simulink subsystem "subsystem_feedbackLinearization"  (R2022a)
settings: Solver=VariableStepAuto  StartTime=0.0  StopTime=10.0  RelTol=1e-3
settings Model: Creator=Philipp  LastModifiedBy=Philipp
settings DebuggingCC: UnconnectedInputMsg=warning  UnconnectedOutputMsg=warning  UnconnectedLineMsg=warning
settings RTWCC: DLArmComputeVersion=19.05

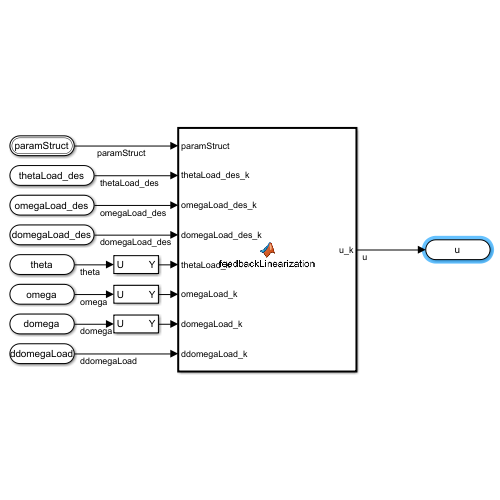
[thumbnail: Simulink's stored preview of the top-level diagram]
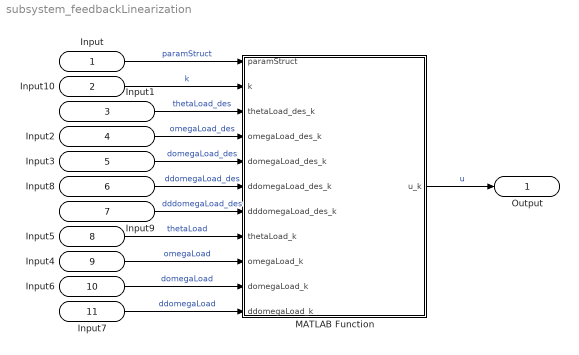
== system subsystem_feedbackLinearization ==
  Input : Inport  OutDataTypeStr=Bus: main_bus
  Input10 : Inport  Port=2
  Input1 : Inport  Port=3
  Input2 : Inport  Port=4
  Input3 : Inport  Port=5
  Input8 : Inport  Port=6
  Input9 : Inport  Port=7
  Input5 : Inport  Port=8
  Input4 : Inport  Port=9
  Input6 : Inport  Port=10
  Input7 : Inport  Port=11
  MATLAB Function : MATLAB Function  TreatAsAtomicUnit=on
  Output : Outport
  wires:
  MATLAB Function/1(u_k) -> Output/1  "u"
  Input/1 -> MATLAB Function/1(paramStruct)  "paramStruct"
  Input1/1 -> MATLAB Function/3(thetaLoad_des_k)  "thetaLoad_des"
  Input2/1 -> MATLAB Function/4(omegaLoad_des_k)  "omegaLoad_des"
  Input3/1 -> MATLAB Function/5(domegaLoad_des_k)  "domegaLoad_des"
  Input5/1 -> MATLAB Function/8(thetaLoad_k)  "thetaLoad"
  Input4/1 -> MATLAB Function/9(omegaLoad_k)  "omegaLoad"
  Input6/1 -> MATLAB Function/10(domegaLoad_k)  "domegaLoad"
  Input7/1 -> MATLAB Function/11(ddomegaLoad_k)  "ddomegaLoad"
  Input8/1 -> MATLAB Function/6(ddomegaLoad_des_k)  "ddomegaLoad_des"
  Input9/1 -> MATLAB Function/7(dddomegaLoad_des_k)  "dddomegaLoad_des"
  Input10/1 -> MATLAB Function/2(k)  "k"

== matlab function subsystem_feedbackLinearization/MATLAB Function ==
  data: paramStruct input; k input; u_k output; thetaLoad_des_k input; omegaLoad_des_k input; domegaLoad_des_k input; ddomegaLoad_des_k input; dddomegaLoad_des_k input; thetaLoad_k input; omegaLoad_k input; domegaLoad_k input; ddomegaLoad_k input
function u_k = feedbackLinearization(paramStruct, k, thetaLoad_des_k, omegaLoad_des_k, domegaLoad_des_k, ddomegaLoad_des_k, dddomegaLoad_des_k, thetaLoad_k, omegaLoad_k, domegaLoad_k, ddomegaLoad_k)

u_k = ...
    feedbackLinearization_model(paramStruct, k, thetaLoad_des_k, omegaLoad_des_k, domegaLoad_des_k, ddomegaLoad_des_k, dddomegaLoad_des_k, thetaLoad_k, omegaLoad_k, domegaLoad_k, ddomegaLoad_k);
